simulink model "Open_Loop_Model_Simulink"  (R2019a)
settings: Solver=VariableStepAuto  StartTime=0.0  StopTime=900  RelTol=1e-3
values from neighbouring files (symbols this model uses):
  c = 1.0791e-5    (= 1.0791e-05)    [Initial_Parameters.m]
  J = J_motor + (J_robot)*(1/G)^2    (= 3.96043)    [Initial_Parameters.m]
  ke = 50.68*60/(2*pi*1000)    (= 0.483958350954)    [Initial_Parameters.m]
  km = 0.415    [Initial_Parameters.m]
  L = 4.8*1e-3    (= 0.0048)    [Initial_Parameters.m]
  R = 9.65    [Initial_Parameters.m]
  V = 12    [Initial_Parameters.m]
settings Model: Creator=sp_ja  LastModifiedBy=sp_ja

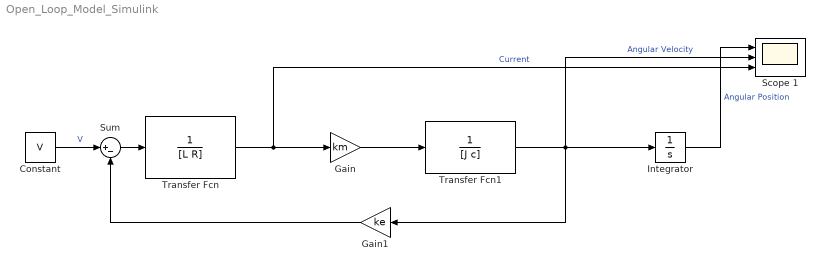
== system Open_Loop_Model_Simulink ==
  "  Scope 1" : Scope  NumInputPorts=3
  Constant : Constant  Value=V
  "Gain " : Gain  Gain=km
  "Gain1 " : Gain  Gain=ke
  "Integrator " : Integrator
  Sum : Sum  Inputs=|+-
  "Transfer Fcn " : TransferFcn  Denominator=[L R]
  "Transfer Fcn1 " : TransferFcn  Denominator=[J c]
  wires:
  Sum/1 -> "Transfer Fcn "/1
  "Gain "/1 -> "Transfer Fcn1 "/1
  "Transfer Fcn "/1 -> "  Scope 1"/3, "Gain "/1  "Current"
  "Transfer Fcn1 "/1 -> "  Scope 1"/2, "Integrator "/1, "Gain1 "/1  "Angular Velocity"
  "Gain1 "/1 -> Sum/2
  Constant/1 -> Sum/1  "V"
  "Integrator "/1 -> "  Scope 1"/1  "Angular Position"
